simulink model "mavlink_gps"  (Simulink 7.5)
settings: Solver=FixedStepDiscrete  SolverMode=SingleTasking  StartTime=0.0  StopTime=10.0  FixedStep=0.001  RelTol=1e-3
undefined symbols (not defined in the file): cpInitCommunications, Init_Reset, MavLinkInit, MavLinkSendHeartbeat, MavLinkSendRawGps, MavLinkSendStatus
libraries: dsPICdrivers x8, simulink x2
settings Model: Creator=Bryant  LastModifiedBy=Bryant
settings OptimizationCC: OptimizeModelRefInitCode=on  LifeSpan=1
settings HardwareCC: ProdBitPerInt=16  ProdEndianess=LittleEndian  ProdWordSize=16  ProdHWDeviceType=16-bit Generic
settings RTWCC: SystemTargetFile=dspic.tlc  MakeCommand=make_CreateMPLAB  TemplateMakefile=dspic_pic30_gcc.tmf  PostCodeGenCommand=dsPIC_Compile()  Description=Embedded Target for Microchip dsPIC (real-time)  ProcessScript=dspic_make_rtw_hook
settings RTWCC: CustomInclude=|
  | ../../mavlink/include
  | ../../clib
settings RTWCC: CustomSource=|
  | ../../clib/mavlink.c
  | ../../clib/uart1.c
  | ../../clib/uart2.c
  | ../../clib/commProtocol.c
  | ../../clib/circBuffer.c
settings CodeAppCC: IgnoreCustomStorageClasses=off
settings STFCustomTargetCC: IncludeMdlTerminateFcn=off  CombineOutputUpdateFcns=on  SuppressErrorStatus=on  ERTCustomFileBanners=on  SupportContinuousTime=off  SupportNonInlinedSFcns=off  SystemTargetFile=dspic.tlc
settings ERTTargetCC: MultiwordLength=2048  ParMdlRefBuildCompliant=off  CompOptLevelCompliant=off  IncludeMdlTerminateFcn=off  SuppressErrorStatus=on  ERTFirstTimeCompliant=off  ModelStepFunctionPrototypeControlCompliant=off  CPPClassGenCompliant=off  ExtModeMexFile=ext_serial_win32_comm  InlinedParameterPlacement=NonHierarchical  ERTSrcFileBannerTemplate=dsPIC_code_template.cgt  ERTHdrFileBannerTemplate=dsPIC_code_template.cgt  ERTDataSrcFileTemplate=dsPIC_code_template.cgt  ERTDataHdrFileTemplate=dsPIC_code_template.cgt  ERTCustomFileTemplate=dsPIC_main.tlc  ConvertIfToSwitch=off
settings CustomProperty: DataType=string  Value=C:\PROGRA~1\MATLAB\R2010a\bin\win64\gmake

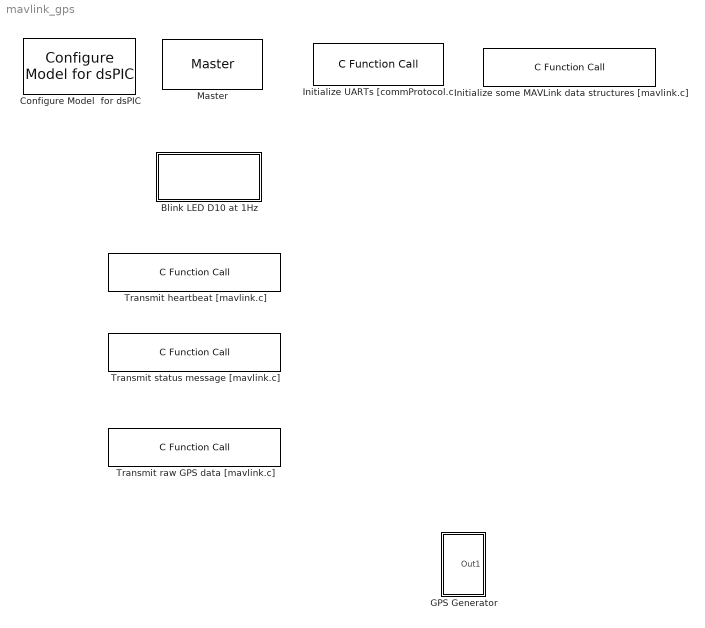
== system mavlink_gps ==
  Blink LED D10 at 1Hz : Subsystem
      mask Display: disp('blink');
  Configure Model  for dsPIC : dsPICdrivers/Simulink Configuration/Configure Model  for dsPIC
  GPS Generator : Subsystem
  Initialize UARTs [commProtocol.c] : dsPICdrivers/OTHERS/C Function Call  Tag=dsPIC_dsPIC_CFunctionCall  FctUpdate=None  fctName=cpInitCommunications  INPUT_SIZE=1  INPUT1=--  INPUT2=--  INPUT3=--  OUTPUT_SIZE=1  OUTPUT1=--  SampleTime=Inf  InputType=[]  OutputType=[]  FctDeclaration=extern void cpInitCommunications();  FctCall=cpInitCommunications();  OrderingInOutPopup=None  FctStart=Start Function (Call once and only once)  FctStart_Name=cpInitCommunications  FctStart_Declaration=inline extern void cpInitCommunications();  FctStart_Call=cpInitCommunications();  FctInit=None  FctInit_Name=Init_Reset  FctInit_Declaration=inline extern void Init_Reset();  FctInit_Call=Init_Reset();  PinDigitalInput=[]  PinDigitalOutput=[]  AnalogueInput=[]
  Initialize some MAVLink data structures [mavlink.c] : dsPICdrivers/OTHERS/C Function Call  Tag=dsPIC_dsPIC_CFunctionCall  FctUpdate=None  fctName=MavLinkSendHeartbeat  INPUT_SIZE=1  INPUT1=--  INPUT2=--  INPUT3=--  OUTPUT_SIZE=1  OUTPUT1=--  SampleTime=1  InputType=[]  OutputType=[]  FctDeclaration=extern void MavLinkSendHeartbeat();  FctCall=MavLinkSendHeartbeat();  OrderingInOutPopup=None  FctStart=Start Function (Call once and only once)  FctStart_Name=MavLinkInit  FctStart_Declaration=inline extern void MavLinkInit();  FctStart_Call=MavLinkInit();  FctInit=None  FctInit_Name=Init_Reset  FctInit_Declaration=inline extern void Init_Reset();  FctInit_Call=Init_Reset();  PinDigitalInput=[]  PinDigitalOutput=[]  AnalogueInput=[]
  Master : dsPICdrivers/Master  Tag=dsPIC_MASTER  Priority=1  TimeStepType=Timer1  picType=33fJ256GP710A  fcy=40000000  Quartz_33f=8e6  PLLActive_33f=on  fcyDesired_33f=40000000  tmr1="[1  39999  0]"  tmr1Info="Time Step : 0.001  ;   Error : 0%  PR1=39999"  tmr2345="[0  0  0  0  0  0  0  0]"  tmr2345cfg=[-1 -1 -1 -1 -1 -1 -1 -1]  IOautoConf=on  typePort="[ 0   0   0   0   0   0   0  10   0   0   0   0   0   0   0   0   0   0   0   0   0   0   0   0   0   0   0   0   0   0   0   0   0   0   0   0   0   0   0   0   0   0   0   0   0   0   0   0   0   0   0   0   0   0   0   0   0   0   0   0   0   0   0   0   0   0   0   0   0   0   0   0   0   0   0   0   0   0   0   0   0   0   0   0   0   0   0   0   0   0   0   0   0   0   0   0   0   0   0   0   0   0   0   0   0   0   0   0   0   0   0   0 ]"  TRIS="[ 65407  65535  65535  65535  65535  65535  65535 ]"  ADPCFG=8388608  MasterBusyPort=None  MasterOverloadPort=None  FOSC=Quartz (XT - HS)  ClockSwitchMonitor=Both disabled  TempProtection_33f=TEMP_ON  FPBOR=<empty>  PWRT=disable  MCLR=<empty>  ICD=ICS_PGD1  JTAGEN=JTAGEN_OFF  PowerSave=off  OverrideFcy=off  NewFcy=1e6  PR2345="[65535  65535  65535  65535  65535  65535  65535  65535]"
  Transmit heartbeat [mavlink.c] : dsPICdrivers/OTHERS/C Function Call  Tag=dsPIC_dsPIC_CFunctionCall  FctUpdate=Output Function  fctName=MavLinkSendHeartbeat  INPUT_SIZE=1  INPUT1=--  INPUT2=--  INPUT3=--  OUTPUT_SIZE=1  OUTPUT1=--  SampleTime=1  InputType=[ ]  OutputType=[ ]  FctDeclaration=extern void MavLinkSendHeartbeat();  FctCall=MavLinkSendHeartbeat();  OrderingInOutPopup=None  FctStart=None  FctStart_Name=cpInitCommunications  FctStart_Declaration=inline extern void cpInitCommunications();  FctStart_Call=cpInitCommunications();  FctInit=None  FctInit_Name=Init_Reset  FctInit_Declaration=inline extern void Init_Reset();  FctInit_Call=Init_Reset();  PinDigitalInput=[]  PinDigitalOutput=[]  AnalogueInput=[]
  Transmit raw GPS data [mavlink.c] : dsPICdrivers/OTHERS/C Function Call  Tag=dsPIC_dsPIC_CFunctionCall  FctUpdate=Output Function  fctName=MavLinkSendRawGps  INPUT_SIZE=1  INPUT1=--  INPUT2=--  INPUT3=--  OUTPUT_SIZE=1  OUTPUT1=--  SampleTime=1  InputType=[ ]  OutputType=[ ]  FctDeclaration=extern void MavLinkSendRawGps();  FctCall=MavLinkSendRawGps();  OrderingInOutPopup=None  FctStart=None  FctStart_Name=cpInitCommunications  FctStart_Declaration=inline extern void cpInitCommunications();  FctStart_Call=cpInitCommunications();  FctInit=None  FctInit_Name=Init_Reset  FctInit_Declaration=inline extern void Init_Reset();  FctInit_Call=Init_Reset();  PinDigitalInput=[]  PinDigitalOutput=[]  AnalogueInput=[]
  Transmit status message [mavlink.c] : dsPICdrivers/OTHERS/C Function Call  Tag=dsPIC_dsPIC_CFunctionCall  FctUpdate=Output Function  fctName=MavLinkSendStatus  INPUT_SIZE=1  INPUT1=--  INPUT2=--  INPUT3=--  OUTPUT_SIZE=1  OUTPUT1=--  SampleTime=1  InputType=[ ]  OutputType=[ ]  FctDeclaration=extern void MavLinkSendStatus();  FctCall=MavLinkSendStatus();  OrderingInOutPopup=None  FctStart=None  FctStart_Name=cpInitCommunications  FctStart_Declaration=inline extern void cpInitCommunications();  FctStart_Call=cpInitCommunications();  FctInit=None  FctInit_Name=Init_Reset  FctInit_Declaration=inline extern void Init_Reset();  FctInit_Call=Init_Reset();  PinDigitalInput=[]  PinDigitalOutput=[]  AnalogueInput=[]

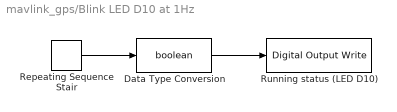
== system mavlink_gps/Blink LED D10 at 1Hz ==
  Data Type Conversion : DataTypeConversion  OutDataTypeMode=boolean  OutDataType=sfix(16)  OutScaling=2^0  OutDataTypeStr=boolean  RndMeth=Simplest
  Repeating Sequence Stair : simulink/Sources/Repeating Sequence Stair  SystemSampleTime=-1  OutValues=[1 0]  tsamp=1  OutMin=[]  OutMax=[]  OutDataTypeStr=double  OutputDataTypeScalingMode=double  OutDataType=fixdt(0,8)  ConRadixGroup=Best Precision: Vector-wise  OutScaling=2^-12
  Running status (LED D10) : dsPICdrivers/Digital I//O/Digital Output Write  Tag=dsPIC_Digital_Output  Priority=5  PORT=A  Pin=[7]  Simultaneous=off  OrderingInOutPopup=None
  wires:
  Repeating Sequence Stair/1 -> Data Type Conversion/1
  Data Type Conversion/1 -> Running status (LED D10)/1

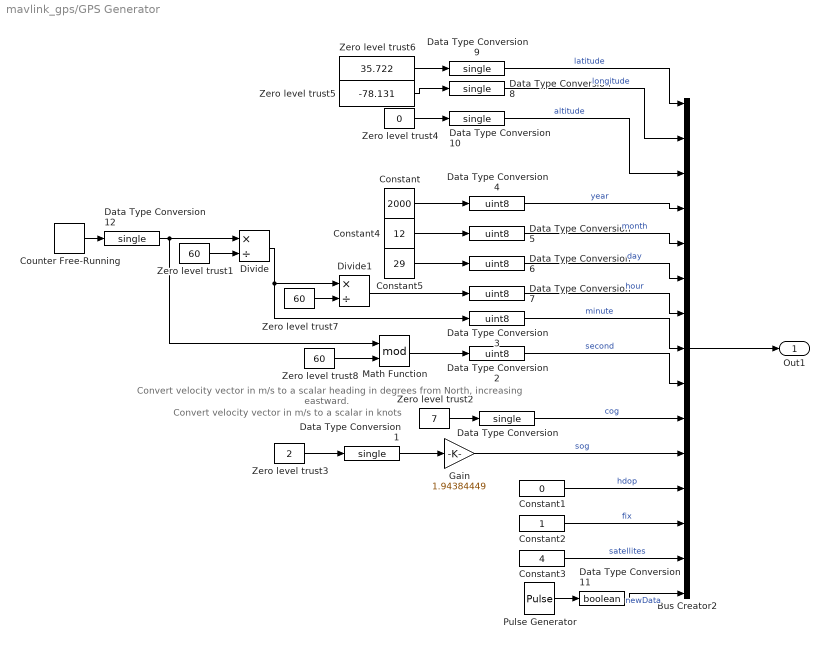
== system mavlink_gps/GPS Generator ==
  note: Convert velocity vector in m/s to a scalar in knots
  note: Convert velocity vector in m/s to a scalar heading in degrees from North, increasing eastward.
  Bus Creator2 : BusCreator  Inputs=15
  Constant : Constant  Value=2000  OutDataTypeMode=uint16  OutDataType=sfix(16)  OutScaling=2^0  OutDataTypeStr=uint16
  Constant1 : Constant  Value=0  OutDataTypeMode=single  OutDataType=fixdt(1, 16)  OutScaling=2^0  OutDataTypeStr=single
  Constant2 : Constant  OutDataTypeMode=uint8  OutDataType=fixdt(1, 16)  OutScaling=2^0  OutDataTypeStr=uint8
  Constant3 : Constant  Value=4  OutDataTypeMode=uint8  OutDataType=fixdt(1, 16)  OutScaling=2^0  OutDataTypeStr=uint8
  Constant4 : Constant  Value=12  OutDataTypeMode=uint16  OutDataType=sfix(16)  OutScaling=2^0  OutDataTypeStr=uint16
  Constant5 : Constant  Value=29  OutDataTypeMode=uint16  OutDataType=sfix(16)  OutScaling=2^0  OutDataTypeStr=uint16
  Counter Free-Running : simulink/Sources/Counter Free-Running  SystemSampleTime=-1  NumBits=16  tsamp=-1
  Data Type Conversion{,1,8..10,12} (6 alike) : DataTypeConversion  OutDataTypeMode=single  OutDataType=fixdt(1, 16)  OutScaling=2^0  OutDataTypeStr=single
  Data Type Conversion11 : DataTypeConversion  OutDataTypeMode=boolean  OutDataType=fixdt(1, 16)  OutScaling=2^0  OutDataTypeStr=boolean
  Data Type Conversion{2..7} (6 alike) : DataTypeConversion  OutDataTypeMode=uint8  OutDataType=fixdt(1, 16)  OutScaling=2^0  OutDataTypeStr=uint8
  Divide : Product  Inputs=*/  OutDataType=fixdt(1, 16)  OutScaling=2^-10
  Divide1 : Product  Inputs=*/  OutDataType=fixdt(1, 16)  OutScaling=2^-10
  Gain : Gain  Gain=1.94384449  ParameterDataType=fixdt(1, 16)  ParameterScaling=2^0  OutDataType=fixdt(1, 16)  OutScaling=2^0
  Math Function : Math  Operator=mod  OutDataType=fixdt(1, 16)  OutScaling=2^0  SaturateOnIntegerOverflow=on
  Pulse Generator : DiscretePulseGenerator  Amplitude=1  Period=100  PulseWidth=1  PhaseDelay=100  SampleTime=.01
  Zero level trust1 : Constant  Value=60  OutDataTypeMode=single  OutDataType=sfix(16)  OutScaling=2^0  OutDataTypeStr=single
  Zero level trust2 : Constant  Value=7  OutDataType=sfix(16)  OutScaling=2^0
  Zero level trust3 : Constant  Value=2  OutDataType=sfix(16)  OutScaling=2^0
  Zero level trust4 : Constant  Value=0  OutDataType=sfix(16)  OutScaling=2^0
  Zero level trust5 : Constant  Value=-78.131  OutDataType=sfix(16)  OutScaling=2^0
  Zero level trust6 : Constant  Value=35.722  OutDataType=sfix(16)  OutScaling=2^0
  Zero level trust7 : Constant  Value=60  OutDataTypeMode=single  OutDataType=sfix(16)  OutScaling=2^0  OutDataTypeStr=single
  Zero level trust8 : Constant  Value=60  OutDataTypeMode=single  OutDataType=sfix(16)  OutScaling=2^0  OutDataTypeStr=single
  Out1 : Outport
  wires:
  Zero level trust6/1 -> Data Type Conversion9/1
  Zero level trust5/1 -> Data Type Conversion8/1
  Zero level trust3/1 -> Data Type Conversion1/1
  Zero level trust2/1 -> Data Type Conversion/1
  Constant/1 -> Data Type Conversion4/1
  Data Type Conversion/1 -> Bus Creator2/10  "cog"
  Data Type Conversion1/1 -> Gain/1
  Data Type Conversion2/1 -> Bus Creator2/9  "second"
  Data Type Conversion3/1 -> Bus Creator2/8  "minute"
  Data Type Conversion4/1 -> Bus Creator2/4  "year"
  Data Type Conversion5/1 -> Bus Creator2/5  "month"
  Data Type Conversion6/1 -> Bus Creator2/6  "day"
  Data Type Conversion7/1 -> Bus Creator2/7  "hour"
  Gain/1 -> Bus Creator2/11  "sog"
  Data Type Conversion8/1 -> Bus Creator2/2  "longitude"
  Data Type Conversion9/1 -> Bus Creator2/1  "latitude"
  Data Type Conversion10/1 -> Bus Creator2/3  "altitude"
  Zero level trust4/1 -> Data Type Conversion10/1
  Constant1/1 -> Bus Creator2/12  "hdop"
  Constant2/1 -> Bus Creator2/13  "fix"
  Constant3/1 -> Bus Creator2/14  "satellites"
  Pulse Generator/1 -> Data Type Conversion11/1
  Data Type Conversion11/1 -> Bus Creator2/15  "newData"
  Bus Creator2/1 -> Out1/1
  Zero level trust1/1 -> Divide/2
  Constant4/1 -> Data Type Conversion5/1
  Constant5/1 -> Data Type Conversion6/1
  Counter Free-Running/1 -> Data Type Conversion12/1
  Divide/1 -> Data Type Conversion3/1, Divide1/1
  Divide1/1 -> Data Type Conversion7/1
  Zero level trust7/1 -> Divide1/2
  Math Function/1 -> Data Type Conversion2/1
  Zero level trust8/1 -> Math Function/2
  Data Type Conversion12/1 -> Divide/1, Math Function/1
